simulink model "Submarine"  (R2025a)
settings: Solver=ode8  StartTime=0.0  StopTime=100  FixedStep=0.01  RelTol=1e-3
libraries: slpidlib x1
settings Model: Creator=aayus  LastModifiedBy=aayus

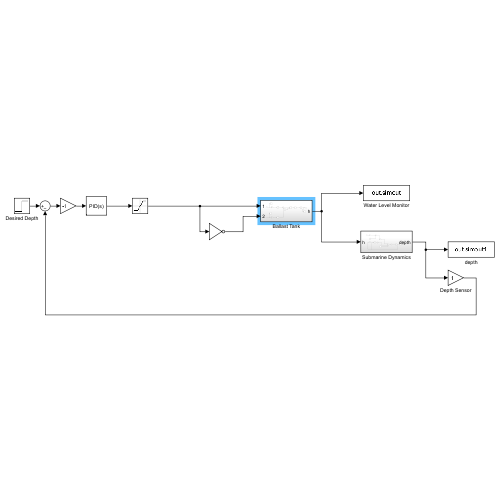
[thumbnail: Simulink's stored preview of the top-level diagram]
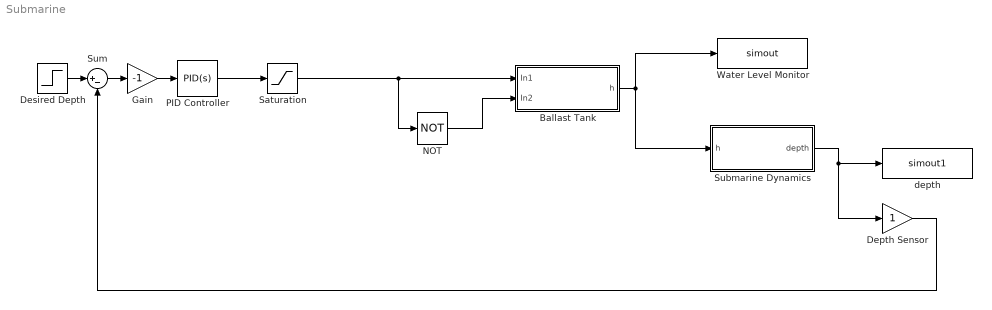
== system Submarine ==
  Ballast Tank : Subsystem
  Depth Sensor : Gain
  Desired Depth : Step  Time=0  After=10  SampleTime=0
  Gain : Gain  Gain=-1
  NOT : Logic  Operator=NOT  IconShape=distinctive  AllPortsSameDT=off  OutDataTypeStr=boolean
  PID Controller : slpidlib/PID Controller  Controller=PID  Form=Parallel  TimeDomain=Continuous-time  UseExternalTs=off  SampleTime=-1  IntegratorMethod=Forward Euler  FilterMethod=Forward Euler  ControllerParametersSource=internal  P=0.1  I=0.01  UseKiTs=off  D=0.5  UseExternalDerivativeSource=off  N=100  UseFilter=on  TunerSelectOption=Transfer Function Based (PID Tuner App)  InitialConditionSource=internal  InitialConditionForIntegrator=0  InitialConditionForFilter=0  DifferentiatorICPrevScaledInput=0  ExternalReset=none  TrackingMode=off  Kt=1  LimitOutput=off  SatLimitsSource=internal  UpperSaturationLimit=inf  LowerSaturationLimit=-inf  LinearizeAsGain=on  AntiWindupMode=none  Kb=1  LimitIntegrator=off  UpperIntegratorSaturationLimit=inf  LowerIntegratorSaturationLimit=-inf  POutMin=[]  POutMax=[]  IOutMin=[]  IOutMax=[]  DOutMin=[]  DOutMax=[]  NOutMin=[]  NOutMax=[]  SumOutMin=[]  SumOutMax=[]  SaturationOutMin=[]  SaturationOutMax=[]  PParamMin=[]  PParamMax=[]  IParamMin=[]  IParamMax=[]  DParamMin=[]  DParamMax=[]  NParamMin=[]  NParamMax=[]  KbParamMin=[]  KbParamMax=[]  KtParamMin=[]  KtParamMax=[]  KbOutMin=[]  KbOutMax=[]  KtOutMin=[]  KtOutMax=[]  IntegratorOutMin=[]  IntegratorOutMax=[]  FilterOutMin=[]  FilterOutMax=[]  SumI1OutMin=[]  SumI1OutMax=[]  SumI2OutMin=[]  SumI2OutMax=[]  SumI3OutMin=[]  SumI3OutMax=[]  SumI4OutMin=[]  SumI4OutMax=[]  SumDOutMin=[]  SumDOutMax=[]  DifferentiatorOutMin=[]  DifferentiatorOutMax=[]  FilterDiffOutCoefMin=[]  FilterDiffOutCoefMax=[]  ReciprocalOutMin=[]  ReciprocalOutMax=[]  SumDenOutMin=[]  SumDenOutMax=[]  SumNumOutMin=[]  SumNumOutMax=[]  DivideOutMin=[]  DivideOutMax=[]  UdiffTsProdOutMin=[]  UdiffTsProdOutMax=[]  NTsProdOutMin=[]  NTsProdOutMax=[]  UintegralTsProdOutMin=[]  UintegralTsProdOutMax=[]  UngainTsProdOutMin=[]  UngainTsProdOutMax=[]  ClampingZeroOutDataTypeStr=Inherit: Inherit via back propagation  ClampingZeroOutMin=[]  ClampingZeroOutMax=[]  FilterDenConstantOutDataTypeStr=Inherit: Inherit via back propagation  FilterDenConstantOutMin=[]  FilterDenConstantOutMax=[]  PCopyOutDataTypeStr=Inherit: Inherit via back propagation  PCopyOutMin=[]  PCopyOutMax=[]  NCopyOutDataTypeStr=Inherit: Inherit via back propagation  NCopyOutMin=[]  NCopyOutMax=[]  IntegratorContinuousStateAttributes=''  IntegratorStateMustResolveToSignalObject=off  IntegratorRTWStateStorageClass=Auto  FilterContinuousStateAttributes=''  FilterStateMustResolveToSignalObject=off  FilterRTWStateStorageClass=Auto  ParallelPVariant=InternalParameters  IdealPVariant=Disabled  IVariant=InternalParameters  DVariant=InternalParameters  IntegratorVariant=Continuous  SatVariant=Disabled  AWVariant=Passthrough  PCopyVariant=Disabled  TRVariant=Disabled  FdbkBlocksVariant=Forward  IdealPFdbkVariant=Disabled  SatFdbkVariant=Disabled  DerivativeFilterVariant=ContFilter  NVariant=InternalParameters  NCopyVariant=Disabled  FilterICVariant=InternalICsFilter  IntegratorICVariant=InternalICs  ExternalResetVariant=Disabled  TRSumVariant=Passthrough  SumFdbkVariant=Disabled  SumVariant=Sum_PID  TsampFilterVariant=InternalTs  TsampNgainVariant=Passthrough  TsampIntegralVariant=Disabled_SignalSpec  ExternalSaturationOutDataTypeStr=Inherit: Same as second input  DerivativeSourceVariant=ErrorSignal  PreIntVariant=InternalPreInt
  Saturation : Saturate  UpperLimit=10  LowerLimit=-10
  Submarine Dynamics : Subsystem
  Sum : Sum  Inputs=|+-
  Water Level Monitor : ToWorkspace  VariableName=simout  SaveFormat=Timeseries  SampleTime=-1
  depth : ToWorkspace  VariableName=simout1  SaveFormat=Timeseries  SampleTime=-1
  wires:
  PID Controller/1 -> Saturation/1
  NOT/1 -> Ballast Tank/2(In2)
  Ballast Tank/1(h) -> Submarine Dynamics/1(h), Water Level Monitor/1
  Submarine Dynamics/1(depth) -> Depth Sensor/1, depth/1
  Desired Depth/1 -> Sum/1
  Sum/1 -> Gain/1
  Depth Sensor/1 -> Sum/2
  Saturation/1 -> NOT/1, Ballast Tank/1(In1)
  Gain/1 -> PID Controller/1

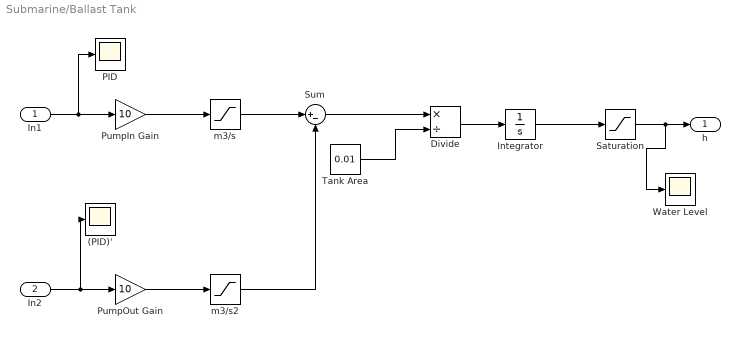
== system Submarine/Ballast Tank ==
  In1 : Inport
  In2 : Inport  Port=2
  (PID)' : Scope
      settings: ActiveDisplayYMinimum=-1  ActiveDisplayYMaximum=1  DataLoggingVariableName=ScopeData2
  Divide : Product  Inputs=*/
  Integrator : Integrator  InitialCondition=0.5
  PID : Scope
      settings: ActiveDisplayYMinimum=-11.121750482256754  ActiveDisplayYMaximum=0.095754340310791
  PumpIn Gain : Gain  Gain=10
  PumpOut Gain : Gain  Gain=10
  Saturation : Saturate  UpperLimit=1  LowerLimit=0
  Sum : Sum  Inputs=|+-
  Tank Area : Constant  Value=0.01
  Water Level : Scope
      settings: ActiveDisplayYMinimum=-703.02596441994638  ActiveDisplayYMaximum=-551.41058755608015
  m3/s : Saturate  UpperLimit=0.0625  LowerLimit=0
  m3/s2 : Saturate  UpperLimit=0.0625  LowerLimit=0  OutDataTypeStr=double
  h : Outport
  wires:
  In1/1 -> PID/1, PumpIn Gain/1
  Sum/1 -> Divide/1
  PumpIn Gain/1 -> m3/s/1
  PumpOut Gain/1 -> m3/s2/1
  Tank Area/1 -> Divide/2
  Divide/1 -> Integrator/1
  Integrator/1 -> Saturation/1
  In2/1 -> (PID)'/1, PumpOut Gain/1
  Saturation/1 -> Water Level/1, h/1
  m3/s/1 -> Sum/1
  m3/s2/1 -> Sum/2

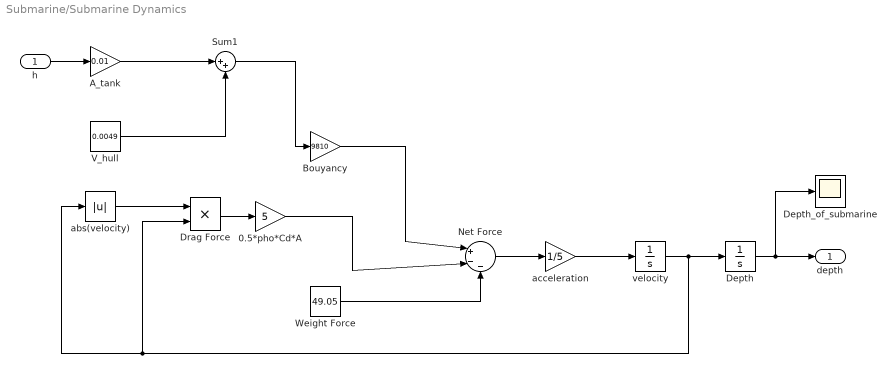
== system Submarine/Submarine Dynamics ==
  h : Inport
  0.5*pho*Cd*A : Gain  Gain=5
  A_tank : Gain  Gain=0.01
  Bouyancy : Gain  Gain=9810
  Depth : Integrator
  Depth_of_submarine : Scope
      settings: ActiveDisplayYMinimum=-49.051487250151339  ActiveDisplayYMaximum=5.4501652500168145  DataLoggingVariableName=ScopeData3
  Drag Force : Product
  Net Force : Sum  Inputs=|+--
  Sum1 : Sum  Inputs=|++
  V_hull : Constant  Value=0.0049
  Weight Force : Constant  Value=49.05
  abs(velocity) : Abs  SaturateOnIntegerOverflow=off
  acceleration : Gain  Gain=1/5
  velocity : Integrator
  depth : Outport
  wires:
  A_tank/1 -> Sum1/1
  V_hull/1 -> Sum1/2
  abs(velocity)/1 -> Drag Force/1
  Bouyancy/1 -> Net Force/1
  0.5*pho*Cd*A/1 -> Net Force/2
  Weight Force/1 -> Net Force/3
  Net Force/1 -> acceleration/1
  acceleration/1 -> velocity/1
  velocity/1 -> Drag Force/2, abs(velocity)/1, Depth/1
  h/1 -> A_tank/1
  Sum1/1 -> Bouyancy/1
  Drag Force/1 -> 0.5*pho*Cd*A/1
  Depth/1 -> Depth_of_submarine/1, depth/1
